simulink model "Pedestrian"  (R2024b)
settings: Solver=VariableStepAuto  StartTime=0.0  StopTime=inf  RelTol=1e-3
values from neighbouring files (symbols this model uses):
  C = [1 0 0 0; 0 1 0 0]    [Car_test_UDP.m]    (also in Final_Code_GPS.m; Final_Code_plotting_reset_kalman.m; KalmanFilter.m)
libraries: sim3dautolib x1, sim3dlib x1
settings Model: Creator=The MathWorks, Inc.  LastModifiedBy=ritvi
settings SolverCC: AlgebraicLoopSolver=TrustRegion
settings OptimizationCC: ReuseModelBlockBuffer=off
settings DebuggingCC: UnconnectedInputMsg=warning  UnconnectedOutputMsg=warning  UnconnectedLineMsg=warning  SymbolicDimsDataTypeCodeGenerationDiagnostic=none
settings ModelReferenceCC: EnableRefExpFcnMdlSchedulingChecks=on
settings RTWCC: GPUComputeCapability=3.5  DLArmComputeVersion=19.05

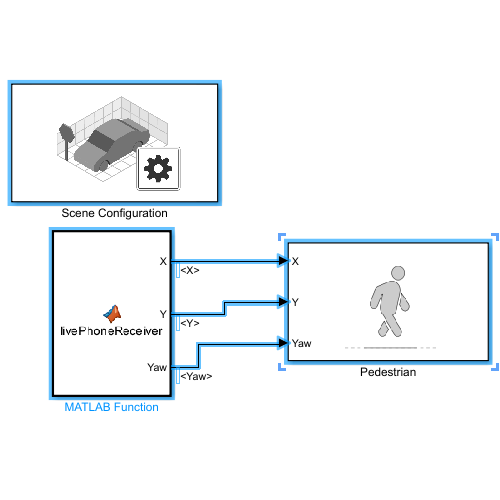
[thumbnail: Simulink's stored preview of the top-level diagram]
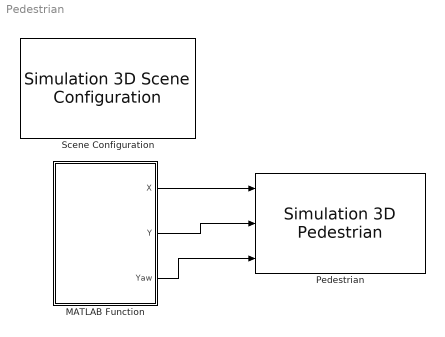
== system Pedestrian ==
  MATLAB Function : MATLAB Function  TreatAsAtomicUnit=on
  Pedestrian : sim3dautolib/Simulation 3D Pedestrian  Priority=-1  PedestrianType=Female 1  Scale=[1, 1, 1]  InitialPos=[50, 50, 0]  InitialYaw=0  ActorName=SimulinkPedestrian1  SampleTime=-1  ActorType=SimulinkPedestrian  ActorTag=SimulinkPedestrian1  ID=1  aMode=3  CoordinateScheme=ISO  TransformOutportEnabled=off
      settings: LibrarySourceBlock=drivingsim3d/Simulation 3D Pedestrian
  Scene Configuration : sim3dlib/Simulation 3D Scene Configuration  Priority=0  ProjectFormat=Unreal Editor  SceneDesc=Large parking lot  ProjectName=C:\Program Files\MATLAB\R2024b\toolbox\shared\sim3d_projects\automotive_project_windows\UE\WindowsNoEditor\VehicleSimulation.exe  ScenePath=/Game/Maps/HwStrght  UEProjPath=C:\Local\AutoVrtlEnv\AutoVrtlEnv.uproject  EnableOpenDRIVE=off  vehTagList={'Custom';'Scene Origin'}  vehTag=Custom  FreeCameraInitialTranslation=[0, 0, 10]  FreeCameraDefaultInitialTranslation=[-6, 0, 2]  FreeCameraInitialRotation=[0, 0, 0]  FreeCameraDefaultInitialRotation=[0, -15, 0]  OpVisEn=off  Ts=1/60  EnableWindow=on  EnableRemoteAccess=off  EnableWeather=off  SunAzimuth=183.600  SunAltitude=0.0  EnableGeospatialSun=off  Latitude=0  Longitude=0  Date=2023-01-01  Time=10:30:00  GeoTimeZone=-5.0  SunDaylightSaving=off  wind=1  clouds=50.0  EnableVolumetricClouds=off  CloudCoverage=0  CloudAltitude=6  fog=0.0  rain=18.0  RaindropsEffect=off  SnowDensity=0  EnableGeospatial=off  UseTrueOrigin=off  OriginHeight=200  OriginLatitude=40.744652  OriginLongitude=-73.988864  MapStyle=Aerial  AdditionalAssetIDs=[]  UseAdvancedSunSky=off  SolarTime=11  TimeZone=-5  Day=21  Month=9  Year=2022  UseDaylightSavingTime=on  DSTStartDay=10  DSTStartMonth=3  DSTEndDay=3  DSTEndMonth=11  DSTSwitchHour=2  sensorTag=MainCamera2  sensorId=2  sensorName=MainCamera2  mountLoc=Origin  offsetFlag=off  tmountOffset=[0, 0, 0]  rmountOffset=[0, 0, 0]  HorizontalResolution=1280  VerticalResolution=720  HorizontalFOV=60  mountPoint=[0 0 0]  mountOrientation=[0 0 0]  aMode=3  ID=2  GeoTrigger=Inactive
      settings: LibrarySourceBlock=drivingsim3d/Simulation 3D Scene Configuration
  wires:
  MATLAB Function/1(X) -> Pedestrian/1
  MATLAB Function/2(Y) -> Pedestrian/2
  MATLAB Function/3(Yaw) -> Pedestrian/3

== matlab function Pedestrian/MATLAB Function ==
  data: X output; Y output; Yaw output
function [X, Y, Yaw] = livePhoneReceiver()
%#codegen
coder.extrinsic('evalin', 'exist');

% 1. Persistent variables ONLY for X and Y smoothing
persistent smooth_X smooth_Y
if isempty(smooth_X)
    smooth_X = 50.0;
    smooth_Y = 50.0;
end

% Pre-allocate variables so Simulink knows their data type (doubles)
target_X = 50.0;
target_Y = 50.0;
target_Yaw = 0.0;

% 2. Check the workspace for the newest target location
if evalin('base', 'exist(''Ped_X'', ''var'')')
    
    target_X   = evalin('base', 'Ped_X');
    target_Y   = evalin('base', 'Ped_Y');
    
    % Grab the pure, unfiltered Yaw directly from the script
    target_Yaw = evalin('base', 'Ped_Yaw');
    
    % --- 3. THE DIGITAL RUBBER BAND (X and Y ONLY) ---
    alpha = 0.15; 
    
    smooth_X = smooth_X + alpha * (target_X - smooth_X);
    smooth_Y = smooth_Y + alpha * (target_Y - smooth_Y);
end

% 4. Output smooth positions, but INSTANT, unfiltered Yaw
X = smooth_X;
Y = smooth_Y;
Yaw = target_Yaw; % <--- Passes straight through!
